simulink model "BLOC_Reference_NEDC"  (R2016a)
settings: Solver=FixedStepDiscrete  StartTime=0.0  StopTime=10.0  FixedStep=hev_dt  RelTol=1e-3
undefined symbols (not defined in the file): dri_cycle_speed_sp, dri_cycle_speed_time, dri_gbx_sp, dri_gbx_time, hev_dt
settings Model: Creator=Florent  LastModifiedBy=Florent
settings OptimizationCC: DefaultParameterBehavior=Inlined  OptimizeModelRefInitCode=on  LifeSpan=1
settings RTWCC: SystemTargetFile=ert.tlc  TemplateMakefile=ert_default_tmf  GenerateReport=on  IncludeHyperlinkInReport=on  LaunchReport=on  TargetLang=C++  GenerateTraceInfo=on  GenerateTraceReport=on  GenerateTraceReportSl=on  GenerateTraceReportSf=on  GenerateTraceReportEml=on
settings CodeAppCC: ForceParamTrailComments=on  OperatorAnnotations=on  SimulinkDataObjDesc=on  SFDataObjDesc=on  MATLABFcnDesc=on  InsertBlockDesc=on  MATLABSourceComments=on
settings ERTTargetCC: GenerateSampleERTMain=on  MultiInstanceERTCode=on  CodeInterfacePackaging=C++ class  SupportContinuousTime=on  InlinedParameterPlacement=NonHierarchical  RootIOFormat=Structure reference  ERTCustomFileTemplate=example_file_process.tlc

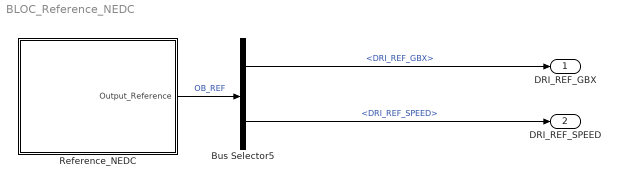
== system BLOC_Reference_NEDC ==
  Bus Selector5 : BusSelector  OutputSignals=DRI_REF_GBX,DRI_REF_SPEED
  Reference_NEDC : Subsystem  TreatAsAtomicUnit=on
  DRI_REF_GBX : Outport
  DRI_REF_SPEED : Outport  Port=2
  wires:
  Bus Selector5/2 -> DRI_REF_SPEED/1  "<DRI_REF_SPEED>"
  Bus Selector5/1 -> DRI_REF_GBX/1  "<DRI_REF_GBX>"
  Reference_NEDC/1(Output_Reference) -> Bus Selector5/1  "OB_REF"

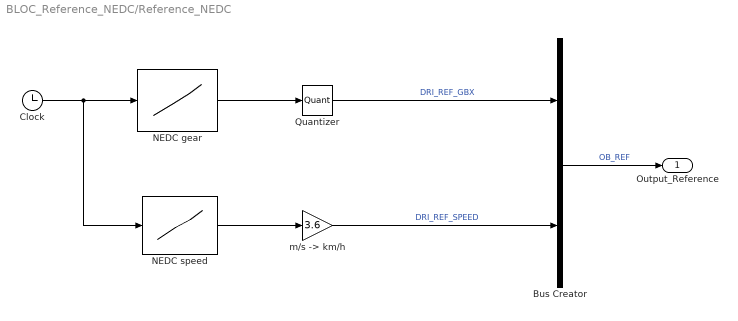
== system BLOC_Reference_NEDC/Reference_NEDC ==
  Bus Creator : BusCreator  Inputs=2
  Clock : Clock
  NEDC gear : Lookup_n-D  NumberOfTableDimensions=1  BreakpointsForDimension1=dri_gbx_time  Table=dri_gbx_sp  InterpMethod=Flat  SampleTime=hev_dt  RndMeth=Simplest  InputSameDT=on
  NEDC speed : Lookup_n-D  NumberOfTableDimensions=1  BreakpointsForDimension1=dri_cycle_speed_time  Table=dri_cycle_speed_sp  SampleTime=hev_dt  RndMeth=Simplest  InputSameDT=on
  Quantizer : Quantizer  QuantizationInterval=1  SampleTime=hev_dt
  "m/s -> km/h" : Gain  Gain=3.6  SampleTime=hev_dt
  Output_Reference : Outport
  wires:
  NEDC gear/1 -> Quantizer/1
  Quantizer/1 -> Bus Creator/1  "DRI_REF_GBX"
  Clock/1 -> NEDC speed/1, NEDC gear/1
  NEDC speed/1 -> "m/s -> km/h"/1
  "m/s -> km/h"/1 -> Bus Creator/2  "DRI_REF_SPEED"
  Bus Creator/1 -> Output_Reference/1  "OB_REF"
